simulink model "MyfirstSimulink"  (Simulink 7.6)
settings: Solver=ode45  StartTime=0.0  StopTime=10.0  RelTol=1e-3
settings Model: Creator=Administrator  LastModifiedBy=Administrator

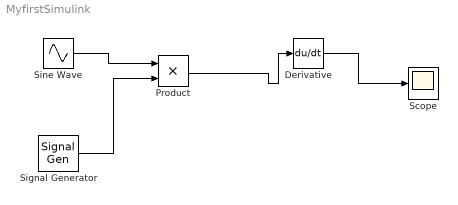
== system MyfirstSimulink ==
  Derivative : Derivative
  Product : Product  RndMeth=Zero
  Scope : Scope
  Signal Generator : SignalGenerator  WaveForm=sawtooth
  Sine Wave : Sin  SampleTime=0
  wires:
  Sine Wave/1 -> Product/1
  Signal Generator/1 -> Product/2
  Product/1 -> Derivative/1
  Derivative/1 -> Scope/1
